simulink subsystem "plant_pid_tuning_ideal"  (R2025b)
settings: Solver=VariableStepAuto  StartTime=0.0  StopTime=10.0  RelTol=1e-3
undefined symbols (not defined in the file or in its folder): do_drag_flag, do_force_flag, do_gravity_flag, do_time_flag, do_torque_flag, drag_wrench, dt_data, I, invI, invM, m, R_cm2cv, rho, V_total, X0
settings Model: Creator=kjhaydon  LastModifiedBy=koryh

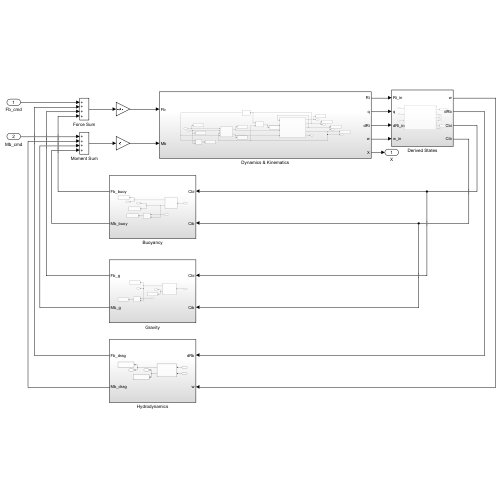
[thumbnail: Simulink's stored preview of the top-level diagram]
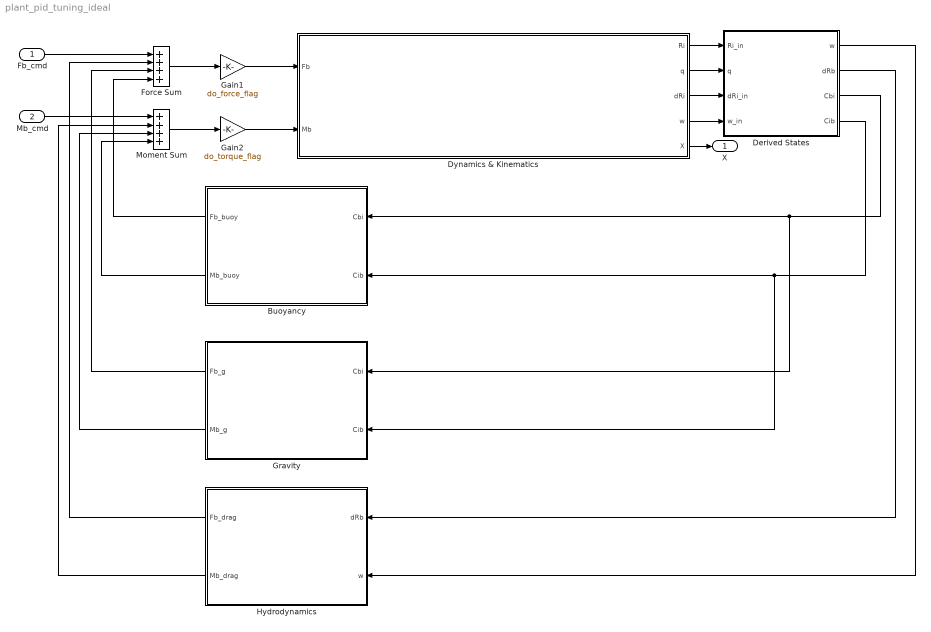
== system plant_pid_tuning_ideal ==
  Fb_cmd : Inport
  Mb_cmd : Inport  Port=2
  Buoyancy : Subsystem
  Derived States : Subsystem
  Dynamics & Kinematics : Subsystem
  Force Sum : Sum  Inputs=++++
  Gain1 : Gain  Gain=do_force_flag
  Gain2 : Gain  Gain=do_torque_flag
  Gravity : Subsystem
  Hydrodynamics : Subsystem
  Moment Sum : Sum  Inputs=++++
  X : Outport
  wires:
  Hydrodynamics/1(Fb_drag) -> Force Sum/2
  Gravity/1(Fb_g) -> Force Sum/3
  Buoyancy/1(Fb_buoy) -> Force Sum/4
  Dynamics & Kinematics/4(w) -> Derived States/4(w_in)
  Dynamics & Kinematics/2(q) -> Derived States/2(q)
  Dynamics & Kinematics/5(X) -> X/1
  Derived States/4(Cib) -> Gravity/2(Cib), Buoyancy/2(Cib)
  Dynamics & Kinematics/1(Ri) -> Derived States/1(Ri_in)
  Derived States/1(w) -> Hydrodynamics/2(w)
  Derived States/2(dRb) -> Hydrodynamics/1(dRb)
  Derived States/3(Cbi) -> Gravity/1(Cbi), Buoyancy/1(Cbi)
  Dynamics & Kinematics/3(dRi) -> Derived States/3(dRi_in)
  Buoyancy/2(Mb_buoy) -> Moment Sum/4
  Hydrodynamics/2(Mb_drag) -> Moment Sum/2
  Gravity/2(Mb_g) -> Moment Sum/3
  Mb_cmd/1 -> Moment Sum/1
  Fb_cmd/1 -> Force Sum/1
  Force Sum/1 -> Gain1/1
  Gain1/1 -> Dynamics & Kinematics/1(Fb)
  Gain2/1 -> Dynamics & Kinematics/2(Mb)
  Moment Sum/1 -> Gain2/1

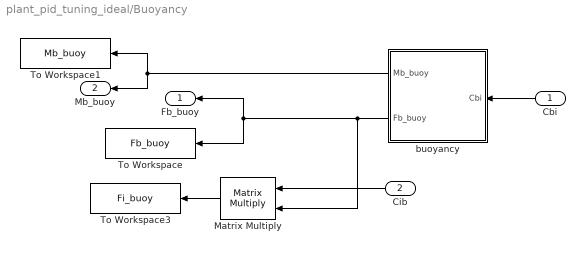
== system plant_pid_tuning_ideal/Buoyancy ==
  Cbi : Inport
  Cib : Inport  Port=2
  Matrix Multiply : Product  Multiplication=Matrix(*)
  To Workspace : ToWorkspace  VariableName=Fb_buoy  SaveFormat=Timeseries  SampleTime=dt_data
  To Workspace1 : ToWorkspace  VariableName=Mb_buoy  SaveFormat=Timeseries  SampleTime=-1
  To Workspace3 : ToWorkspace  VariableName=Fi_buoy  SaveFormat=Timeseries  SampleTime=dt_data
  buoyancy : MATLAB Function  TreatAsAtomicUnit=on
  Fb_buoy : Outport
  Mb_buoy : Outport  Port=2
  wires:
  Cib/1 -> Matrix Multiply/1
  Matrix Multiply/1 -> To Workspace3/1
  Cbi/1 -> buoyancy/1(Cbi)
  buoyancy/1(Mb_buoy) -> To Workspace1/1, Mb_buoy/1
  buoyancy/2(Fb_buoy) -> Matrix Multiply/2, Fb_buoy/1, To Workspace/1

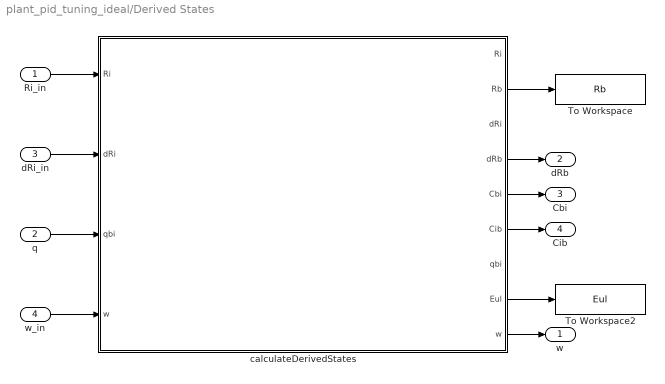
== system plant_pid_tuning_ideal/Derived States ==
  Ri_in : Inport
  q : Inport  Port=2
  dRi_in : Inport  Port=3
  w_in : Inport  Port=4
  To Workspace : ToWorkspace  VariableName=Rb  SaveFormat=Timeseries  SampleTime=dt_data
  To Workspace2 : ToWorkspace  VariableName=Eul  SaveFormat=Timeseries  SampleTime=dt_data
  calculateDerivedStates : MATLAB Function  TreatAsAtomicUnit=on
  w : Outport
  dRb : Outport  Port=2
  Cbi : Outport  Port=3
  Cib : Outport  Port=4
  wires:
  calculateDerivedStates/2(Rb) -> To Workspace/1
  calculateDerivedStates/6(Cib) -> Cib/1
  calculateDerivedStates/4(dRb) -> dRb/1
  calculateDerivedStates/5(Cbi) -> Cbi/1
  calculateDerivedStates/8(Eul) -> To Workspace2/1
  calculateDerivedStates/9(w) -> w/1
  w_in/1 -> calculateDerivedStates/4("w ")
  q/1 -> calculateDerivedStates/3("qbi ")
  dRi_in/1 -> calculateDerivedStates/2("dRi ")
  Ri_in/1 -> calculateDerivedStates/1("Ri ")

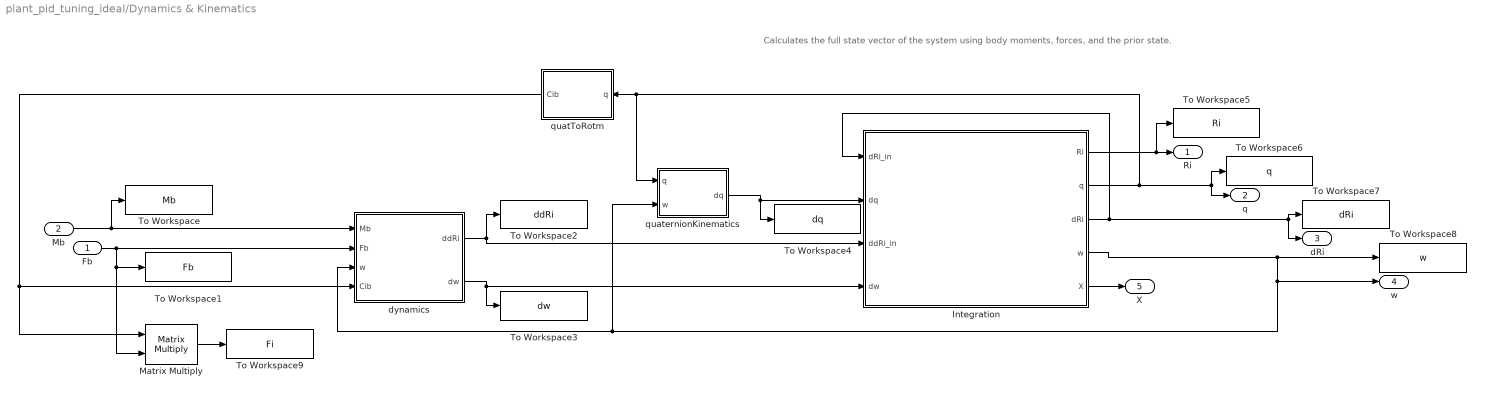
== system plant_pid_tuning_ideal/Dynamics & Kinematics ==
  note: Calculates the full state vector of the system using body moments, forces, and the prior state.
  Fb : Inport
  Mb : Inport  Port=2
  Integration : Subsystem
  Matrix Multiply : Product  Multiplication=Matrix(*)
  To Workspace : ToWorkspace  VariableName=Mb  SaveFormat=Timeseries  SampleTime=dt_data
  To Workspace1 : ToWorkspace  VariableName=Fb  SaveFormat=Timeseries  SampleTime=dt_data
  To Workspace2 : ToWorkspace  VariableName=ddRi  SaveFormat=Timeseries  SampleTime=dt_data
  To Workspace3 : ToWorkspace  VariableName=dw  SaveFormat=Timeseries  SampleTime=dt_data
  To Workspace4 : ToWorkspace  VariableName=dq  SaveFormat=Timeseries  SampleTime=dt_data
  To Workspace5 : ToWorkspace  VariableName=Ri  SaveFormat=Timeseries  SampleTime=dt_data
  To Workspace6 : ToWorkspace  VariableName=q  SaveFormat=Timeseries  SampleTime=dt_data
  To Workspace7 : ToWorkspace  VariableName=dRi  SaveFormat=Timeseries  SampleTime=dt_data
  To Workspace8 : ToWorkspace  VariableName=w  SaveFormat=Timeseries  SampleTime=dt_data
  To Workspace9 : ToWorkspace  VariableName=Fi  SaveFormat=Timeseries  SampleTime=dt_data
  dynamics : MATLAB Function  TreatAsAtomicUnit=on
  quatToRotm : MATLAB Function  TreatAsAtomicUnit=on
  quaternionKinematics : MATLAB Function  TreatAsAtomicUnit=on
  Ri : Outport
  q : Outport  Port=2
  dRi : Outport  Port=3
  w : Outport  Port=4
  X : Outport  Port=5
  wires:
  Integration/5(X) -> X/1
  Matrix Multiply/1 -> To Workspace9/1
  quatToRotm/1(Cib) -> Matrix Multiply/1, dynamics/4(Cib)
  Fb/1 -> dynamics/2(Fb), Matrix Multiply/2, To Workspace1/1
  Mb/1 -> dynamics/1(Mb), To Workspace/1
  dynamics/1(ddRi) -> Integration/3(ddRi_in), To Workspace2/1
  dynamics/2(dw) -> Integration/4(dw), To Workspace3/1
  Integration/3(dRi) -> Integration/1(dRi_in), To Workspace7/1, dRi/1
  Integration/2(q) -> quatToRotm/1(q), quaternionKinematics/1(q), To Workspace6/1, q/1
  Integration/4(w) -> To Workspace8/1, w/1, quaternionKinematics/2(w), dynamics/3(w)
  quaternionKinematics/1(dq) -> Integration/2(dq), To Workspace4/1
  Integration/1(Ri) -> To Workspace5/1, Ri/1

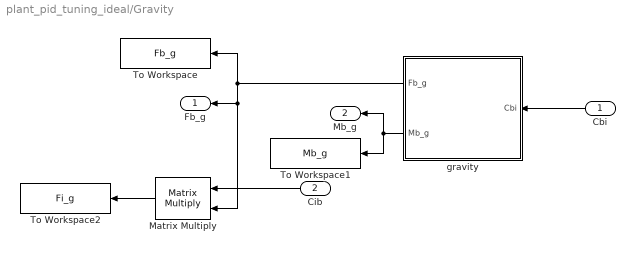
== system plant_pid_tuning_ideal/Gravity ==
  Cbi : Inport
  Cib : Inport  Port=2
  Matrix Multiply : Product  Multiplication=Matrix(*)
  To Workspace : ToWorkspace  VariableName=Fb_g  SaveFormat=Timeseries  SampleTime=dt_data
  To Workspace1 : ToWorkspace  VariableName=Mb_g  SaveFormat=Timeseries  SampleTime=dt_data
  To Workspace2 : ToWorkspace  VariableName=Fi_g  SaveFormat=Timeseries  SampleTime=-1
  gravity : MATLAB Function  TreatAsAtomicUnit=on
  Fb_g : Outport
  Mb_g : Outport  Port=2
  wires:
  Matrix Multiply/1 -> To Workspace2/1
  Cib/1 -> Matrix Multiply/1
  gravity/2(Mb_g) -> Mb_g/1, To Workspace1/1
  Cbi/1 -> gravity/1(Cbi)
  gravity/1(Fb_g) -> To Workspace/1, Matrix Multiply/2, Fb_g/1

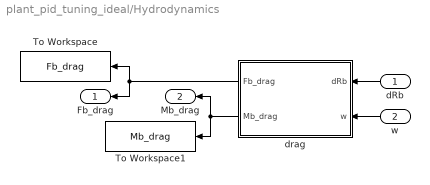
== system plant_pid_tuning_ideal/Hydrodynamics ==
  dRb : Inport
  w : Inport  Port=2
  To Workspace : ToWorkspace  VariableName=Fb_drag  SaveFormat=Timeseries  SampleTime=dt_data
  To Workspace1 : ToWorkspace  VariableName=Mb_drag  SaveFormat=Timeseries  SampleTime=dt_data
  drag : MATLAB Function  TreatAsAtomicUnit=on
  Fb_drag : Outport
  Mb_drag : Outport  Port=2
  wires:
  drag/1(Fb_drag) -> To Workspace/1, Fb_drag/1
  dRb/1 -> drag/1(dRb)
  drag/2(Mb_drag) -> Mb_drag/1, To Workspace1/1
  w/1 -> drag/2(w)

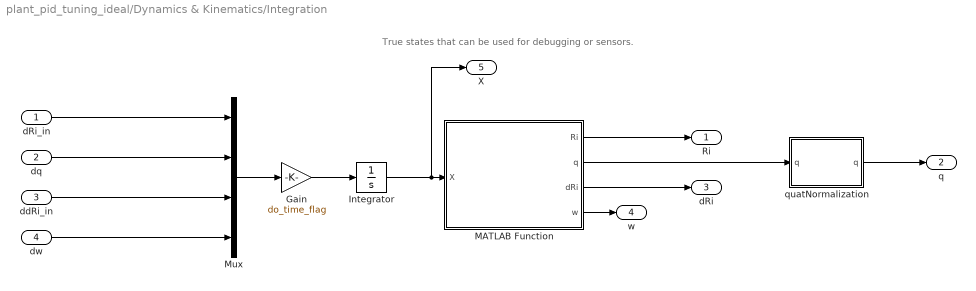
== system plant_pid_tuning_ideal/Dynamics & Kinematics/Integration ==
  note: True states that can be used for debugging or sensors.
  dRi_in : Inport
  dq : Inport  Port=2
  ddRi_in : Inport  Port=3
  dw : Inport  Port=4
  Gain : Gain  Gain=do_time_flag
  Integrator : Integrator  InitialCondition=X0
  MATLAB Function : MATLAB Function  TreatAsAtomicUnit=on
  Mux : Mux
  quatNormalization : MATLAB Function  TreatAsAtomicUnit=on
  Ri : Outport
  q : Outport  Port=2
  dRi : Outport  Port=3
  w : Outport  Port=4
  X : Outport  Port=5
  wires:
  Gain/1 -> Integrator/1
  Mux/1 -> Gain/1
  MATLAB Function/2(q) -> quatNormalization/1("q ")
  quatNormalization/1(q) -> q/1
  Integrator/1 -> MATLAB Function/1(X), X/1
  MATLAB Function/4(w) -> w/1
  MATLAB Function/3(dRi) -> dRi/1
  MATLAB Function/1(Ri) -> Ri/1
  dRi_in/1 -> Mux/1
  dq/1 -> Mux/2
  dw/1 -> Mux/4
  ddRi_in/1 -> Mux/3

== matlab function plant_pid_tuning_ideal/Hydrodynamics/drag ==
  data: dRb input; Fb_drag output; w input; Mb_drag output; drag_wrench parameter; do_drag_flag parameter
function [Fb_drag,Mb_drag] = fcn(dRb, w, drag_wrench, do_drag_flag)

[Fb_drag, Mb_drag] = drag(dRb, w, drag_wrench, do_drag_flag);

== matlab function plant_pid_tuning_ideal/Dynamics & Kinematics/Integration/MATLAB Function ==
  data: X input; Ri output; q output; dRi output; w output
function [Ri,q,dRi,w] = fcn(X)
Ri = X(1:3);
q = X(4:7);
dRi = X(8:10);
w = X(11:13);
end

== matlab function plant_pid_tuning_ideal/Dynamics & Kinematics/dynamics ==
  data: Mb input; ddRi output; Fb input; w input; Cib input; dw output; I parameter; invM parameter; invI parameter
function [ddRi, dw] = fcn(Mb, Fb, w, Cib, I, invM, invI)

[ddRi,dw] = dynamics(Mb,Fb,w,Cib,I,invM,invI);

== matlab function plant_pid_tuning_ideal/Derived States/calculateDerivedStates ==
  data: Ri input; Ri output; dRi input; qbi input; w input; Rb output; dRi output; dRb output; Cbi output; Cib output; qbi output; Eul output; w output
function [Ri,Rb,dRi,dRb,Cbi,Cib,qbi,Eul,w] = fcn(Ri,dRi,qbi,w)

[Ri,Rb,dRi,dRb,Cbi,Cib,qbi,Eul,w] = calculateDerivedStates(Ri,dRi,qbi,w);

== matlab function plant_pid_tuning_ideal/Dynamics & Kinematics/quaternionKinematics ==
  data: q input; dq output; w input
function dq = fcn(q,w)

dq = quaternionKinematics(q,w);

== matlab function plant_pid_tuning_ideal/Dynamics & Kinematics/Integration/quatNormalization ==
  data: q input; q output
function q = fcn(q)

q = quatNormalization(q);

== matlab function plant_pid_tuning_ideal/Dynamics & Kinematics/quatToRotm ==
  data: q input; Cib output
function Cib = fcn(q)

Cib = quatToRotm(q);

== matlab function plant_pid_tuning_ideal/Buoyancy/buoyancy ==
  data: Mb_buoy output; Fb_buoy output; rho parameter; V_total parameter; R_cm2cv parameter; Cbi input
function [Mb_buoy,Fb_buoy] = fcn(rho, V_total, R_cm2cv, Cbi)


[Fb_buoy, Mb_buoy] =  buoyancy(Cbi, rho, V_total, R_cm2cv);

== matlab function plant_pid_tuning_ideal/Gravity/gravity ==
  data: Cbi input; Fb_g output; Mb_g output; m parameter; do_gravity_flag parameter
function [Fb_g, Mb_g] = fcn(Cbi, m, do_gravity_flag)

[Fb_g, Mb_g] = gravity(Cbi, m, do_gravity_flag);
